simulink model "demo1202_smd_io"  (R2015b)
settings: Solver=ode1  SolverMode=SingleTasking  StartTime=0.0  StopTime=Inf  FixedStep=0.0001  RelTol=1e-3
PostLoadFcn:
  | , if any(exist('dsrtsu_mdlpostloadfcn', 'file') == [2, 3, 6]), try dsrtsu_mdlpostloadfcn('Execute', bdroot); catch fprintf('Error in PostLoadFcn (dsrtsu_mdlpostloadfcn) for model "%s":\n %s\n', bdroot, lasterr); end, end,
libraries: rti1202lib_adc_class2 x1, rti1202lib_dac_class1 x1
settings Model: DSRTSU_INTERNAL_RTI_VER=500  DSRTSU_INTERNAL_RTI_TYPE=rti1202  RTICANMMDATA=struct('GeneralSetupData',struct('modelroot',['L:\New folder\REC_Maroje\Demo1\RTI\Demos\Model\DS1202\Model'],'generalsettings',struct('filesettings',struct('destfolder',struct('Name','RTICANMM_FILES','Check',1),'buildfolder',struct('Name','.','Check',1),'AbsDestfolder',struct('Name',['L:\New folder\REC_Maroje\Demo1\RTI\Demos\Model\DS1202\Model\RTICANMM_FILES']),'AbsBuildfolder',struct('Name',['L:\New folder\REC_Maroje\Demo1\RTI\Demos\Model\DS1202\Model']))),'options',struct('addpaths',1,'rmpaths',1,'addtrcexclusion',logical(1),'cannavigator',struct('checkmonitoring',0),'show_usrtrc',0,'use_usrtrc',0),'advanced',struct('options',ones(1,100)),'MPSetup',{{}},'modelname','demo1202_smd_io','block','demo1202_smd_io'))  DSRTSU_INTERNAL_RTIFLEXRAYCONFIG=110  DSRTSU_INTERNAL_RTIFPGA=90  ExtModeTrigMode=oneshot  ExtModeArmWhenConnect=off  Creator=dSPACE GmbH  LastModifiedBy=dSPACE GmbH
settings DataIOCC: SaveFormat=Array  SignalLoggingSaveFormat=ModelDataLogs
settings OptimizationCC: BlockReduction=off  ConditionallyExecuteInputs=off  OptimizeBlockIOStorage=off  BufferReuse=off  GlobalBufferReuse=off  ExpressionFolding=off  ExpressionDepthLimit=2147483647  LocalBlockOutputs=off  InitFltsAndDblsToZero=on
settings DebuggingCC: SaveWithParameterizedLinksMsg=none  UnderspecifiedInitializationDetection=Classic  MergeDetectMultiDrivingBlocksExec=none  SignalResolutionControl=TryResolveAllWithWarning  SolverPrmCheckMsg=warning  MultiTaskDSMMsg=warning  MultiTaskCondExecSysMsg=none  MultiTaskRateTransMsg=warning  TasksWithSamePriorityMsg=none  FcnCallInpInsideContextMsg=UseLocalSettings  StateNameClashWarn=warning  StrictBusMsg=None
settings HardwareCC: ProdBitPerPointer=32  ProdLargestAtomicInteger=Integer  ProdEndianess=BigEndian  ProdWordSize=32  ProdHWDeviceType=Custom Processor->Custom  TargetIntDivRoundTo=Zero  TargetEndianess=BigEndian  TargetHWDeviceType=Custom Processor->Custom
settings RTWCC: SystemTargetFile=rti1202.tlc  MakeCommand=make_rti  TemplateMakefile=rti1202.tmf  Description=dSPACE DS1202 Hardware Platform  RTWVerbose=off
settings STFCustomTargetCC: ParMdlRefBuildCompliant=on  ConcurrentExecutionCompliant=off  GeneratePreprocessorConditionals=Use local settings  CPPClassGenCompliant=off  GRTInterface=off  SystemTargetFile=rti1202.tlc
settings GRTTargetCC: CompOptLevelCompliant=off  ConcurrentExecutionCompliant=off  CombineOutputUpdateFcns=off  MatFileLogging=off  CPPClassGenCompliant=off  UseToolchainInfoCompliant=off  ExtModeMexFile=noextcomm
settings ConfigComp: CovModelRefEnable=Off

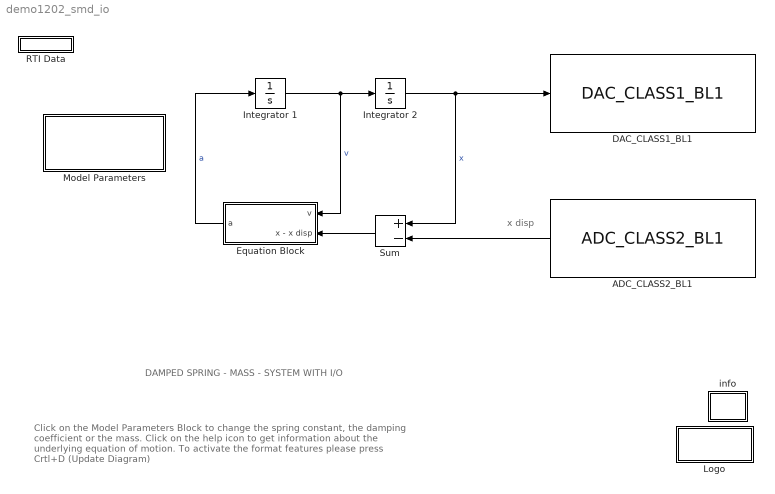
== system demo1202_smd_io ==
  note: DAMPED SPRING - MASS - SYSTEM WITH I/O
  note: Click on the Model Parameters Block to change the spring constant,
      | the damping coefficient or the mass.
      | Click on the help icon to get information about the underlying equation
      | of motion.
      |
      | To activate the format features please press Crtl+D (Update Diagram)
  note: x disp
  ADC_CLASS2_BL1 : rti1202lib_adc_class2/ADC_CLASS2_BL1  DSProperties=struct('RTI',struct('Version',uint32(1),'BlockType',struct('isSLSource',uint8(1),'isSLSink',uint8(1),'isHWSource',uint8(0),'isHWSink',uint8(1),'isSetup',uint8(0),'isInline',uint8(1),'isNonInline',uint8(0),'isInterrupt',uint8(0),'isChannelwise',uint8(1)),'IOBoardType',{{'DS120X','STD','ADCC2'}},'UnitType','ADC','Identifier','ADC','DialogType','ML','BlockSet','NONE','SlaveProcessor','NONE'))  RTIBlockInterface=struct('OutputPortsActive',1,'OutputPortsWidth',int32(1),'OutputPortsDataType',{{'SS_DOUBLE'}},'OutputPortsName',{{'ADC'}},'DialogFcn','rti120xstdadcc2adcgui','InitLevel',3,'IconTransparency','on','BlockDisplay',{{['ADC CL2\nChannel: 1'],'center'}},'BlockName',struct('Token',{{'ADC_CLASS2_BL1'}}))  RTIBlockParameters=struct('ChannelNo',{{1,'OFF',[]}},'TLCFileName',{{'rti120xadc_c2_adc','OFF',[]}})  RTISFcnParameters=struct('ChannelNo','int16','TLCFileName','char')  RTIBlockParaDefault=struct('ChannelNo',1,'TLCFileName','rti120xadc_c2_adc')
  DAC_CLASS1_BL1 : rti1202lib_dac_class1/DAC_CLASS1_BL1  DSProperties=struct('RTI',struct('Version',uint32(2),'BlockType',struct('isSLSource',uint8(0),'isSLSink',uint8(1),'isHWSource',uint8(0),'isHWSink',uint8(1),'isSetup',uint8(0),'isInline',uint8(1),'isNonInline',uint8(0),'isInterrupt',uint8(0),'isChannelwise',uint8(1)),'IOBoardType',{{'DS120X','STD','DACC1'}},'UnitType','DAC','Identifier','DAC','DialogType','ML','BlockSet','NONE','SlaveProcessor','NONE'))  RTIBlockInterface=struct('InputPortsActive',1,'InputPortsWidth',int32(1),'InputPortsDataType',{{'SS_DOUBLE'}},'InputPortsName',{{['DAC 1']}},'DialogFcn','rti120xstddacc1dacgui','InitLevel',3,'IconTransparency','on','BlockDisplay',{{['DAC CL1\nChannel: 1'],'center'}},'BlockName',struct('Token',{{'DAC_CLASS1_BL1'}}))  RTIBlockParameters=struct('ChannelNo',{{1,'OFF',[]}},'ChannelNumOf',{{1,'OFF',[]}},'InitialValue1',{{0,'OFF',[-10 10]}},'InitialValue2',{{0,'OFF',[-10 10]}},'InitialValue3',{{0,'OFF',[-10 10]}},'InitialValue4',{{0,'OFF',[-10 10]}},'InitialValue5',{{0,'OFF',[-10 10]}},'InitialValue6',{{0,'OFF',[-10 10]}},'InitialValue7',{{0,'OFF',[-10 10]}},'InitialValue8',{{0,'OFF',[-10 10]}},'InitialValue9',{{0,'OFF',[-10 10]}},'InitialValue10',{{0,'OFF',[-10 10]}},'InitialValue11',{{0,'OFF',[-10 10]}},'InitialValue12',{{0,'OFF',[-10 10]}},'InitialValue13',{{0,'OFF',[-10 10]}},'InitialValue14',{{0,'OFF',[-10 10]}},'InitialValue15',{{0,'OFF',[-10 10]}},'InitialValue16',{{0,'OFF',[-10 10]}},'TermValue1',{{0,'OFF',[-10 10]}},'TermValue2',{{0,'OFF',[-10 10]}},'TermValue3',{{0,'OFF',[-10 10]}},'TermValue4',{{0,'OFF',[-10 10]}},'TermValue5',{{0,'OFF',[-10 10]}},'TermValue6',{{0,'OFF',[-10 10]}},'TermValue7',{{0,'OFF',[-10 10]}},'TermValue8',{{0,'OFF',[-10 10]}},'TermValue9',{{0,'OFF',[-10 10]}},'TermValue10',{{0,'OFF',[-10 10]}},'TermValue11',{{0,'OFF',[-10 10]}},'TermValue12',{{0,'OFF',[-10 10]}},'TermValue13',{{0,'OFF',[-10 10]}},'TermValue14',{{0,'OFF',[-10 10]}},'TermValue15',{{0,'OFF',[-10 10]}},'TermValue16',{{0,'OFF',[-10 10]}},'TLCFileName',{{'rti120xdac_c1_dac','OFF',[]}},'InitialValueBuildCheck1',{{0,'OFF',[]}},'InitialValueBuildCheck2',{{0,'OFF',[]}},'InitialValueBuildCheck3',{{0,'OFF',[]}},'InitialValueBuildCheck4',{{0,'OFF',[]}},'InitialValueBuildCheck5',{{0,'OFF',[]}},'InitialValueBuildCheck6',{{0,'OFF',[]}},'InitialValueBuildCheck7',{{0,'OFF',[]}},'InitialValueBuildCheck8',{{0,'OFF',[]}},'InitialValueBuildCheck9',{{0,'OFF',[]}},'InitialValueBuildCheck10',{{0,'OFF',[]}},'InitialValueBuildCheck11',{{0,'OFF',[]}},'InitialValueBuildCheck12',{{0,'OFF',[]}},'InitialValueBuildCheck13',{{0,'OFF',[]}},'InitialValueBuildCheck14',{{0,'OFF',[]}},'InitialValueBuildCheck15',{{0,'OFF',[]}},'InitialValueBuildCheck16',{{0,'OFF',[]}},'TermValueBuildCheck1',{{0,'OFF',[]}},'TermValueBuildCheck2',{{0,'OFF',[]}},'TermValueBuildCheck3',{{0,'OFF',[]}},'TermValueBuildCheck4',{{0,'OFF',[]}},'TermValueBuildCheck5',{{0,'OFF',[]}},'TermValueBuildCheck6',{{0,'OFF',[]}},'TermValueBuildCheck7',{{0,'OFF',[]}},'TermValueBuildCheck8',{{0,'OFF',[]}},'TermValueBuildCheck9',{{0,'OFF',[]}},'TermValueBuildCheck10',{{0,'OFF',[]}},'TermValueBuildCheck11',{{0,'OFF',[]}},'TermValueBuildCheck12',{{0,'OFF',[]}},'TermValueBuildCheck13',{{0,'OFF',[]}},'TermValueBuildCheck14',{{0,'OFF',[]}},'TermValueBuildCheck15',{{0,'OFF',[]}},'TermValueBuildCheck16',{{0,'OFF',[]}},'OutputMode',{{ones(1,16),'OFF',[1 2]}},'EnableTermMode',{{1,'OFF',[0 1]}})  RTISFcnParameters=struct('ChannelNo','int16','ChannelNumOf','int16','InitialValue1','double','InitialValue2','double','InitialValue3','double','InitialValue4','double','InitialValue5','double','InitialValue6','double','InitialValue7','double','InitialValue8','double','InitialValue9','double','InitialValue10','double','InitialValue11','double','InitialValue12','double','InitialValue13','double','InitialValue14','double','InitialValue15','double','InitialValue16','double','TermValue1','double','TermValue2','double','TermValue3','double','TermValue4','double','TermValue5','double','TermValue6','double','TermValue7','double','TermValue8','double','TermValue9','double','TermValue10','double','TermValue11','double','TermValue12','double','TermValue13','double','TermValue14','double','TermValue15','double','TermValue16','double','TLCFileName','char','EnableTermMode','int16','OutputMode','int16')  RTIBlockParaDefault=struct('ChannelNo',1,'ChannelNumOf',1,'InitialValue1',0,'InitialValue2',0,'InitialValue3',0,'InitialValue4',0,'InitialValue5',0,'InitialValue6',0,'InitialValue7',0,'InitialValue8',0,'InitialValue9',0,'InitialValue10',0,'InitialValue11',0,'InitialValue12',0,'InitialValue13',0,'InitialValue14',0,'InitialValue15',0,'InitialValue16',0,'TermValue1',0,'TermValue2',0,'TermValue3',0,'TermValue4',0,'TermValue5',0,'TermValue6',0,'TermValue7',0,'TermValue8',0,'TermValue9',0,'TermValue10',0,'TermValue11',0,'TermValue12',0,'TermValue13',0,'TermValue14',0,'TermValue15',0,'TermValue16',0,'TLCFileName','rti120xdac_c1_dac','InitialValueBuildCheck1',0,'InitialValueBuildCheck2',0,'InitialValueBuildCheck3',0,'InitialValueBuildCheck4',0,'InitialValueBuildCheck5',0,'InitialValueBuildCheck6',0,'InitialValueBuildCheck7',0,'InitialValueBuildCheck8',0,'InitialValueBuildCheck9',0,'InitialValueBuildCheck10',0,'InitialValueBuildCheck11',0,'InitialValueBuildCheck12',0,'InitialValueBuildCheck13',0,'InitialValueBuildCheck14',0,'InitialValueBuildCheck15',0,'InitialValueBuildCheck16',0,'TermValueBuildCheck1',0,'TermValueBuildCheck2',0,'TermValueBuildCheck3',0,'TermValueBuildCheck4',0,'TermValueBuildCheck5',0,'TermValueBuildCheck6',0,'TermValueBuildCheck7',0,'TermValueBuildCheck8',0,'TermValueBuildCheck9',0,'TermValueBuildCheck10',0,'TermValueBuildCheck11',0,'TermValueBuildCheck12',0,'TermValueBuildCheck13',0,'TermValueBuildCheck14',0,'TermValueBuildCheck15',0,'TermValueBuildCheck16',0,'EnableTermMode',0,'OutputMode',ones(1,16))
  Equation Block : Subsystem
  Integrator 1 : Integrator
  Integrator 2 : Integrator
  Logo : Subsystem  mask(dSPACE){EmptyParameter=[]}
      mask prompts: EmptyParameter "Mask Parameter 1:"
      settings: OpenFcn=;
      mask Display: image(imread('rti_mdl_dslogo.tif'));
  Model Parameters : Subsystem  mask{C=20000, d=16, m=0.04}
      mask prompts: C "Spring constant : C"; d "Damping coefficient : d"; m "Mass : m"
      mask Display: fprintf('Spring constant : C\nDamping coefficient : d\nMass : m')
  RTI Data : Subsystem  Tag=struct('RTIDataServer',struct('RTIDataServerVs','2','RTIModelDescription','struct(''main'',''demo1202_smd_io'',''sub'','''',''isMp'',0)'))  LoadFcn="if exist('rtidc'), try,  rtidc('DataHostBlockClbLoad', gcbh); catch, disp(['Warning: ''LoadFcn'' for RTI Data block failed: ' lasterr]); end, end,"  mask(RTI_DATA_HOST){}
      mask help:
      | RTI Data Block.
      | This block is used by RTI to store internal model-dependent data.
      | Please keep this block on the root level of the model. Deleting this block will result in data loss.
      |
      | NEVER DELETE OR COPY THIS BLOCK!
      settings: CopyFcn="if exist('rtidc'), try,  rtidc('DataHostBlockClbCopy', gcbh); catch, disp(['Warning: ''CopyFcn'' for RTI Data block failed: ' lasterr]); end, end,"  DeleteFcn="if exist('rtidc'), try,  rtidc('DataHostBlockClbDelete', gcbh); catch, disp(['Warning: ''DeleteFcn'' for RTI Data block failed: ' lasterr]); end, end,"  ModelCloseFcn="if exist('rtidc'), try,  rtidc('DataHostBlockClbModelClose', gcbh); catch, disp(['Warning: ''ModelCloseFcn'' for RTI Data block failed: ' lasterr]); end, end,"  PreSaveFcn="if exist('rtidc'), try,  rtidc('DataHostBlockClbPreSave', gcbh); catch, disp(['Warning: ''PreSaveFcn'' for RTI Data block failed: ' lasterr]); end, end,"  PostSaveFcn="if exist('rtidc'), try,  rtidc('DataHostBlockClbPostSave', gcbh); catch, disp(['Warning: ''PostSaveFcn'' for RTI Data block failed: ' lasterr]); end, end,"  NameChangeFcn="if exist('rtidc'), try,  rtidc('DataHostBlockClbNameChange', gcbh); catch, disp(['Warning: ''NameChangeFcn'' for RTI Data block failed: ' lasterr]); end, end,"
      mask Help:
      | RTI Data Block.
      | This block is used by RTI to store internal model-dependent data.
      | Please keep this block on the root level of the model. Deleting this block will result in data loss.
      | 
      | NEVER DELETE OR COPY THIS BLOCK!
      mask Display:
      | text(0.5, 0.5, 'RTI Data', 'HorizontalAlignment', 'center');
      | plot([1 0]);
  Sum : Sum  Inputs=+-  SaturateOnIntegerOverflow=on  InputSameDT=on  OutDataTypeStr=Inherit: Same as first input
  info : Subsystem
      mask Display: disp('?')
  wires:
  Integrator 1/1 -> Integrator 2/1, Equation Block/1(v)  "v"
  Integrator 2/1 -> DAC_CLASS1_BL1/1, Sum/1  "x"
  Sum/1 -> Equation Block/2(x - x disp)
  Equation Block/1(a) -> Integrator 1/1  "a"
  ADC_CLASS2_BL1/1 -> Sum/2

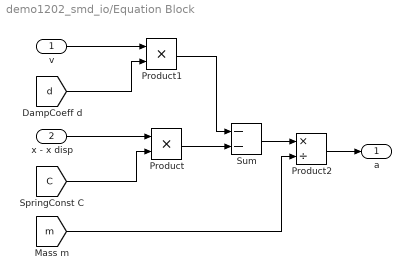
== system demo1202_smd_io/Equation Block ==
  v : Inport
  x - x disp : Inport  Port=2
  Product : Product  SaturateOnIntegerOverflow=on  InputSameDT=on  OutDataTypeStr=Inherit: Same as first input
  Product1 : Product  SaturateOnIntegerOverflow=on  InputSameDT=on  OutDataTypeStr=Inherit: Same as first input
  Product2 : Product  Inputs=*/  SaturateOnIntegerOverflow=on  InputSameDT=on  OutDataTypeStr=Inherit: Same as first input
  Sum : Sum  Inputs=--  SaturateOnIntegerOverflow=on  InputSameDT=on  OutDataTypeStr=Inherit: Same as first input
  a : Outport
  wires:
  x - x disp/1 -> Product/1
  [C] -> Product/2
  v/1 -> Product1/1
  [d] -> Product1/2
  Product1/1 -> Sum/1
  Product/1 -> Sum/2
  Sum/1 -> Product2/1
  [m] -> Product2/2
  Product2/1 -> a/1

== system demo1202_smd_io/Logo ==
  note: $Revision: 2.2 $
  note: $Date: 2012/07/16 15:49:23MESZ $
  note: $RCSfile: demom_smd_io.mdl $

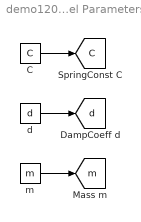
== system demo1202_smd_io/Model Parameters ==
  C : Constant  Value=C
  d : Constant  Value=d
  m : Constant  Value=m
  tag scope: C=global, d=global, m=global
  wires:
  C/1 -> [C]
  d/1 -> [d]
  m/1 -> [m]

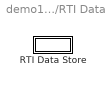
== system demo1202_smd_io/RTI Data ==
  RTI Data Store : Subsystem  Tag="struct('private',struct('version',struct('dsVer',uint32(2),'dsVerCreation',uint32(2),'RTI',struct('ver','3.6.0b5','type','RTI1003')),'access',struct('type','Model','isPerm',1,'created',['22-Sep-2000 15:35:44'],'modified',['03-Feb-2017 15:09:04'],'location','')),'public',struct('main',struct('data',[]),'sub',struct('name',{{'demo1202_smd_io'}},'data',{{struct('TH',struct('thTaskInfo',struct('taskType',{'TIMER','HWINT','TMRINT','SWINT','GLINT'},'tasksNumOf',{1,0,0,0,0},'srcIds',{{'TIMERA'},{},{},{},{}},'taskNames',{{['Timer Task 1']},{},{},{},{}})),'th_tc',struct('dataType','TASK','taskGroupId','','taskGroupList',{{}},'taskSchedulingPolicy','FCFS','taskType','TIMER','blkh',-1,'srcId','TIMERA','srcSgnName',['Timer A interrupt'],'srcCpuName','','taskName',['Timer Task 1  [0.0001] s'],'taskNameDisplayExt','','smplTime',0.0001,'smplTimeOffs',0,'hasFixedPriority',0,'priority',1,'hasFixedOvc',0,'ovcType',1,'ovcMax',0),'tc_th',struct('dataType','TASK','taskGroupId','','taskGroupList',{{}},'taskSchedulingPolicy','FCFS','taskType','TIMER','blkh',-1,'srcId','TIMERA','srcSgnName',['Timer A interrupt'],'srcCpuName','','taskName',['Timer Task 1  [0.0001] s'],'taskNameDisplayExt','','smplTime',0.0001,'smplTimeOffs',0,'hasFixedPriority',0,'priority',1,'hasFixedOvc',0,'ovcType',1,'ovcMax',0))}})))"  mask(RTI_DATA_STORE){}
      mask help:
      | RTI Data Store Block. This block is used by RTI to store internal model dependent data. Deleting this block will result in data loss.
      |
      | NEVER DELETE, COPY, OR MODIFY THIS BLOCK!
      mask Help:
      | RTI Data Store Block. This block is used by RTI to store internal model dependent data. Deleting this block will result in data loss.
      | 
      | NEVER DELETE, COPY, OR MODIFY THIS BLOCK!
      mask Display: text(0.5, 0.5, ' ', 'HorizontalAlignment', 'center');

== system demo1202_smd_io/info ==
  note: a
      | d
      | m
      | v
      | C
      | x
      | x disp
      | f
      | t
      | u
  note: This demo example illustrates the behavior of a damped Spring-Mass-System.
      | After downloading the model to the DS1202, use ControlDesk NG to change the model para-
      | meters and to view the results.
      |
      | The equation of motion for the center of the mass driven by an external force is:
      |
      | a   =  -  (d / m) * v  -  (C / m)*( x - x disp )
  note: : acceleration of mass
      | : damping coeffecient
      | : mass
      | : velocity of the mass
      | : spring constant
      | : position of mass
      | : excitation
      | : frequency
      | : time
      | : amplitude of excitation
  note: The output of the Integrator 1 is v and is multiplied with d / m in the equation block.
      | The output x of the Integrator 2 can be measured on DAC channel 1. It  is added to x disp,
      | and the sum is multiplied with C / m in the equation block.
      | The output of the ADC is the exciting displacement of the mass:  x disp.
      |
      | In the case of a sine-like excitation the driving force is:
      | F = x disp * C
      | x disp  = u * cos ( 2pi * f * t)
      | The solution of the equation of motion is:
      | x ( t ) = xo * cos (2pi * f * t - alpha)
      | a harmonic oscillation with the original frequency, an amplitude xo and a phase alpha,
      | both depending on the model parameters.
      |
      | In the case of a square-like excitation the driving force results from a single displacement
      | of u, twice in the period T = 1 / f :
      | F = u * C
      | The solution of the equation of motion is:
      | x ( t ) = xo * exp[ - (d / 2m)* t ] * cos ( omega * t )
      | an exponentially decreasing sine wave with the natural frequency:
      | omega = sqrt [ (C / m) - ( d^2 / 4 m^2) ]
  note: MODEL DEMO1202_SMD_IO
  note: [m/s^2]
      | [kg/s]
      | [kg]
      | [m/s]
      | [kg/s^2]
      | [m]
      | [m]
      | [Hz]
      | [s]
      | [m]
  note: .

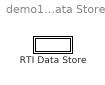
== system demo1202_smd_io/RTI Data/RTI Data Store ==
  RTI Data Store : Subsystem  mask(RTI_DATA_STORE){}
      mask help:
      | RTI Data Store Block. This block is used by RTI to store internal model dependent data. Deleting this block will result in data loss.
      |
      | NEVER DELETE, COPY, OR MODIFY THIS BLOCK!
      mask Help:
      | RTI Data Store Block. This block is used by RTI to store internal model dependent data. Deleting this block will result in data loss.
      | 
      | NEVER DELETE, COPY, OR MODIFY THIS BLOCK!
      mask Display: text(0.5, 0.5, ' ', 'HorizontalAlignment', 'center');

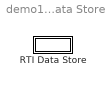
== system demo1202_smd_io/RTI Data/RTI Data Store/RTI Data Store ==
  RTI Data Store : Subsystem  mask(RTI_DATA_STORE){}
      mask help:
      | RTI Data Store Block. This block is used by RTI to store internal model dependent data. Deleting this block will result in data loss.
      |
      | NEVER DELETE, COPY, OR MODIFY THIS BLOCK!
      mask Help:
      | RTI Data Store Block. This block is used by RTI to store internal model dependent data. Deleting this block will result in data loss.
      | 
      | NEVER DELETE, COPY, OR MODIFY THIS BLOCK!
      mask Display: text(0.5, 0.5, ' ', 'HorizontalAlignment', 'center');

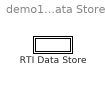
== system demo1202_smd_io/RTI Data/RTI Data Store/RTI Data Store/RTI Data Store ==
  RTI Data Store : Subsystem  mask(RTI_DATA_STORE){}
      mask help:
      | RTI Data Store Block. This block is used by RTI to store internal model dependent data. Deleting this block will result in data loss.
      |
      | NEVER DELETE, COPY, OR MODIFY THIS BLOCK!
      mask Help:
      | RTI Data Store Block. This block is used by RTI to store internal model dependent data. Deleting this block will result in data loss.
      | 
      | NEVER DELETE, COPY, OR MODIFY THIS BLOCK!
      mask Display: text(0.5, 0.5, ' ', 'HorizontalAlignment', 'center');

== system demo1202_smd_io/RTI Data/RTI Data Store/RTI Data Store/RTI Data Store/RTI Data Store ==
